simulink model "sistema"  (R2018a)
settings: Solver=VariableStepAuto  StartTime=0.0  StopTime=10.0  RelTol=1e-3
values from neighbouring files (symbols this model uses):
  wn = 8.036118730219977    (= 8.03611873022)    [entrada_arbitraria.m]    (also in entrada_arbitrária.m; parametros_pid.m; teste_aleatorio_input.m; teste_bw.m = 1)
  zeta = 0.900733958553509    (= 0.900733958554)    [entrada_arbitraria.m]    (also in entrada_arbitrária.m; parametros_pid.m; teste_aleatorio_input.m; teste_bw.m = 1)
libraries: simulink x1
settings Model: Creator=Eric Moretti  LastModifiedBy=Eric Moretti

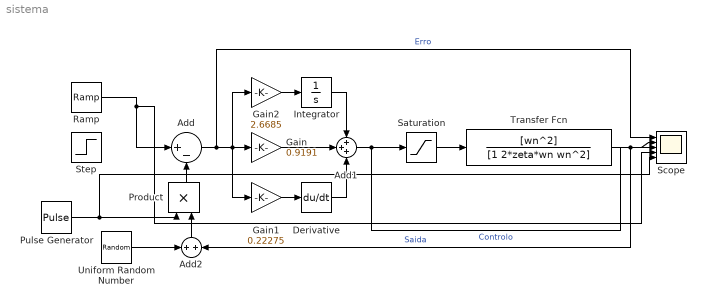
== system sistema ==
  Add : Sum  Inputs=|+-
  Add1 : Sum  Inputs=+++
  Add2 : Sum  Inputs=+|+
  Derivative : Derivative
  Gain : Gain  Gain=0.9191
  Gain1 : Gain  Gain=0.22275
  Gain2 : Gain  Gain=2.6685
  Integrator : Integrator
  Product : Product
  Pulse Generator : DiscretePulseGenerator  PulseType=Time based  Period=5  PulseWidth=50
  Ramp : simulink/Sources/Ramp  slope=-0.1  start=0  InitialOutput=1
  Saturation : Saturate  UpperLimit=1  LowerLimit=0
  Scope : Scope  NumInputPorts=5
  Step : Step  Time=0  SampleTime=0
  Transfer Fcn : TransferFcn  Numerator=[wn^2]  Denominator=[1 2*zeta*wn wn^2]
  Uniform Random Number : UniformRandomNumber  Minimum=-0.001  Maximum=0.001  SampleTime=0.1
  wires:
  Transfer Fcn/1 -> Add2/2, Scope/2  "Saida"
  Add1/1 -> Scope/3, Saturation/1  "Controlo"
  Derivative/1 -> Add1/3
  Gain1/1 -> Derivative/1
  Gain/1 -> Add1/2
  Gain2/1 -> Integrator/1
  Integrator/1 -> Add1/1
  Add/1 -> Scope/1, Gain1/1, Gain2/1, Gain/1  "Erro"
  Uniform Random Number/1 -> Add2/1
  Add2/1 -> Product/2
  Product/1 -> Add/2
  Pulse Generator/1 -> Scope/5, Product/1
  Saturation/1 -> Transfer Fcn/1
  Ramp/1 -> Scope/4, Add/1
